simulink model "board_unspecific_RTOS_blinky"  (R2016b)
settings: Solver=FixedStepDiscrete  StartTime=0.0  StopTime=10.0  FixedStep=1e-3  RelTol=1e-3
libraries: mbed_lib x3, simulink x1
settings Model: MbedPath=E:\GitSynology\mbed_target\targets\NUCLEO_F303RE  Creator=oh  LastModifiedBy=oh
settings DataIOCC: LimitDataPoints=on  SaveFormat=Array
settings OptimizationCC: LifeSpan=1
settings DebuggingCC: SolverPrmCheckMsg=warning  SFUnexpectedBacktrackingDiag=warning  SFNoUnconditionalDefaultTransitionDiag=warning  SFExecutionAtInitializationDiag=none
settings HardwareCC: ProdBitPerPointer=32  ProdBitPerSizeT=32  ProdBitPerPtrDiffT=32  ProdLargestAtomicInteger=Long  ProdLargestAtomicFloat=Double  ProdIntDivRoundTo=Undefined  ProdWordSize=32  ProdHWDeviceType=ARM Compatible->ARM Cortex
settings ModelReferenceCC: PropagateSignalLabelsOutOfModel=off
settings RTWCC: SystemTargetFile=mbed.tlc  TemplateMakefile=mbed.tmf  Description=Mbed Target (Embedded Target)  TargetLang=C++
settings CodeAppCC: IgnoreCustomStorageClasses=off
settings STFCustomTargetCC: TargetLibSuffix=.a  GenerateSampleERTMain=on  CombineOutputUpdateFcns=on  ERTCustomFileBanners=on  SupportContinuousTime=off  SupportNonInlinedSFcns=off  RemoveResetFunc=on  MATLABClassNameForMDSCustomization=Simulink.SoftwareTarget.ERTCustomization  GRTInterface=off  SystemTargetFile=mbed.tlc
settings ERTTargetCC: GenerateSampleERTMain=on  ParMdlRefBuildCompliant=off  CompOptLevelCompliant=off  ConcurrentExecutionCompliant=off  ERTFirstTimeCompliant=off  ModelStepFunctionPrototypeControlCompliant=off  CPPClassGenCompliant=off  UseToolchainInfoCompliant=off  ERTCustomFileTemplate=mbed_file_process.tlc  ConvertIfToSwitch=off  SuppressUnreachableDefaultCases=off
settings ConfigComp: CovMetricSettings=dw  CovHtmlReporting=on  CovSaveCumulativeToWorkspaceVar=on  CovSaveSingleToWorkspaceVar=on  CovExternalEMLEnable=off  CovSFcnEnable=off

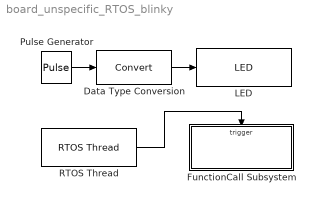
== system board_unspecific_RTOS_blinky ==
  Data Type Conversion : DataTypeConversion
  FunctionCall Subsystem : Subsystem  TreatAsAtomicUnit=on
  LED : mbed_lib/GPIO/LED  nLED=1  SampleTime=-1
  Pulse Generator : DiscretePulseGenerator  PulseType=Time based  Period=1  PulseWidth=50
  RTOS Thread : mbed_lib/RTOS/RTOS Thread  ThreadPriority=Normal  StackOption=Default  StackSize=1024  Timing=500
  wires:
  Pulse Generator/1 -> Data Type Conversion/1
  Data Type Conversion/1 -> LED/1
  RTOS Thread/1 -> FunctionCall Subsystem/Trigger

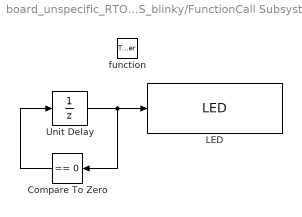
== system board_unspecific_RTOS_blinky/FunctionCall Subsystem ==
  function : TriggerPort  TriggerType=function-call  VariantControl=Variant
  Compare To Zero : simulink/Logic and Bit Operations/Compare To Zero  relop===  OutDataTypeStr=uint8
  LED : mbed_lib/GPIO/LED  nLED=2  SampleTime=-1
  Unit Delay : UnitDelay  SampleTime=-1
  wires:
  Unit Delay/1 -> LED/1, Compare To Zero/1
  Compare To Zero/1 -> Unit Delay/1
